simulink model "model"  (R2023a)
settings: Solver=VariableStepAuto  StartTime=0.0  StopTime=10.0  RelTol=1e-6
values from neighbouring files (symbols this model uses):
  a1 = a1_nom    (= 5)    [main.m]
  a2 = a2_nom    (= 1)    [main.m]
  k = acker(A,b,p)    [main.m]
  kn = 1./(-c/(A-b*k)*b)    [main.m]
  l = acker(A',c',pl)    [main.m]
  x0 = i    [main.m]
settings Model: Creator=User  LastModifiedBy=User

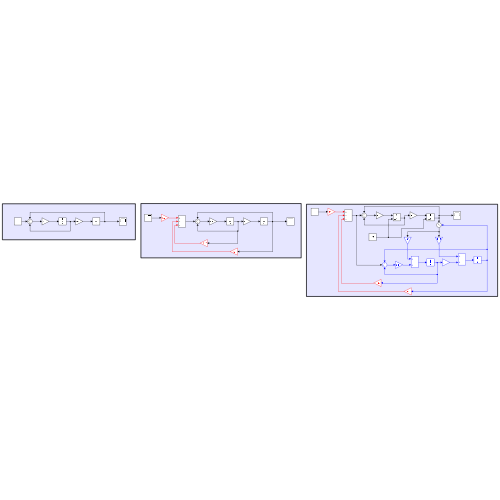
[thumbnail: Simulink's stored preview of the top-level diagram]
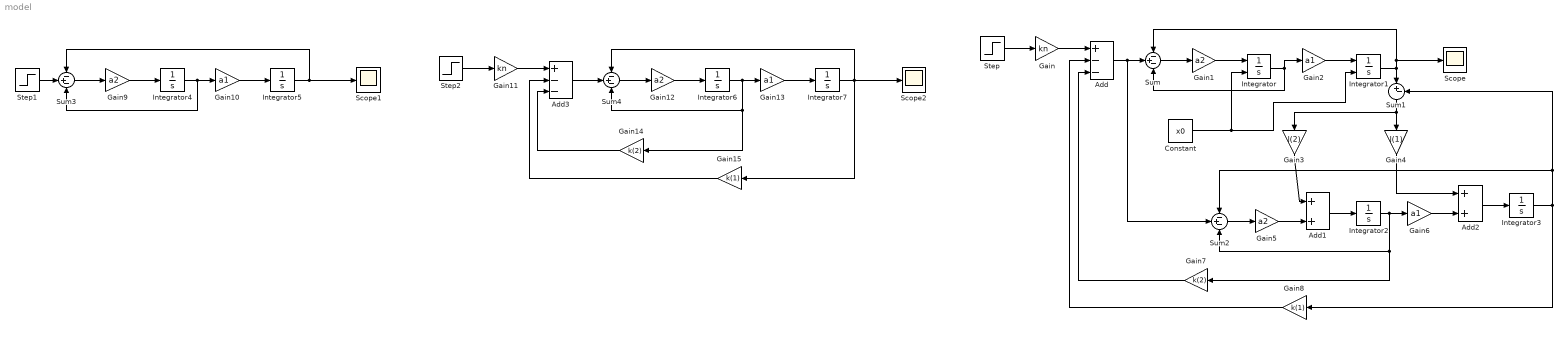
== system model ==
  Add : Sum  Inputs=+--
  Add1 : Sum
  Add2 : Sum
  Add3 : Sum  Inputs=+--
  Constant : Constant  Value=x0
  Gain : Gain  Gain=kn
  Gain{1,5,9,12} (4 alike) : Gain  Gain=a2
  Gain{2,6,10,13} (4 alike) : Gain  Gain=a1
  Gain11 : Gain  Gain=kn
  Gain14 : Gain  Gain=k(2)
  Gain15 : Gain  Gain=k(1)
  Gain3 : Gain  Gain=l(2)
  Gain4 : Gain  Gain=l(1)
  Gain7 : Gain  Gain=k(2)
  Gain8 : Gain  Gain=k(1)
  Integrator : Integrator  InitialConditionSource=external
  Integrator1 : Integrator  InitialConditionSource=external
  Integrator{2..7} (6 alike) : Integrator
  Scope : Scope
  Scope1 : Scope
  Scope2 : Scope
  Step : Step  Time=0  SampleTime=0
  Step1 : Step  Time=0  SampleTime=0
  Step2 : Step  Time=0  SampleTime=0
  Sum{,2..4} (4 alike) : Sum  Inputs=-+-
  Sum1 : Sum  Inputs=|+-
  wires:
  Step/1 -> Gain/1
  Gain/1 -> Add/1
  Add/1 -> Sum2/2, Sum/2
  Sum/1 -> Gain1/1
  Gain1/1 -> Integrator/1
  Integrator/1 -> Gain2/1, Sum/3
  Gain2/1 -> Integrator1/1
  Integrator1/1 -> Scope/1, Sum/1, Sum1/1
  Sum1/1 -> Gain3/1, Gain4/1
  Add1/1 -> Integrator2/1
  Integrator2/1 -> Gain7/1, Sum2/3, Gain6/1
  Gain6/1 -> Add2/2
  Gain4/1 -> Add2/1
  Gain5/1 -> Add1/2
  Add2/1 -> Integrator3/1
  Gain3/1 -> Add1/1
  Sum2/1 -> Gain5/1
  Integrator3/1 -> Sum1/2, Sum2/1, Gain8/1
  Gain7/1 -> Add/3
  Gain8/1 -> Add/2
  Step1/1 -> Sum3/2
  Gain9/1 -> Integrator4/1
  Sum3/1 -> Gain9/1
  Integrator4/1 -> Sum3/3, Gain10/1
  Integrator5/1 -> Scope1/1, Sum3/1
  Gain10/1 -> Integrator5/1
  Gain14/1 -> Add3/3
  Gain12/1 -> Integrator6/1
  Add3/1 -> Sum4/2
  Step2/1 -> Gain11/1
  Sum4/1 -> Gain12/1
  Integrator6/1 -> Gain14/1, Sum4/3, Gain13/1
  Integrator7/1 -> Gain15/1, Scope2/1, Sum4/1
  Gain13/1 -> Integrator7/1
  Gain15/1 -> Add3/2
  Gain11/1 -> Add3/1
  Constant/1 -> Integrator/2, Integrator1/2
